simulink model "Example_2_Integral_Control_Mdl"  (Simulink 7.1)
settings: Solver=ode23s  StartTime=0.0  StopTime=5  RelTol=1e-3
values from neighbouring files (symbols this model uses):
  A = sys.a    [Example_2_Control.m]    (also in Example_2_Discretization.m; Example_2_Disturbance_Estimation.m; Example_2_Integral_Control.m; Example_2_Prediction_Observer.m)
  a_ramp = 0.05    [Example_2_Control.m]    (also in Example_2_Discretization.m; Example_2_Integral_Control.m; Example_2_Prediction_Observer.m; Example_2_Reduced_Order_Observer.m)
  a_sin = 0.1    [Example_2_Control.m]    (also in Example_2_Discretization.m; Example_2_Integral_Control.m; Example_2_Prediction_Observer.m; Example_2_Reduced_Order_Observer.m)
  B = sys.b    [Example_2_Control.m]    (also in Example_2_Discretization.m; Example_2_Disturbance_Estimation.m; Example_2_Integral_Control.m; Example_2_Prediction_Observer.m)
  B_w = sys_d.b    [Example_2_Control.m]    (also in Example_2_Discretization.m; Example_2_Disturbance_Estimation.m; Example_2_Integral_Control.m; Example_2_Prediction_Observer.m)
  C = sys.c    [Example_2_Control.m]    (also in Example_2_Discretization.m; Example_2_Disturbance_Estimation.m; Example_2_Integral_Control.m; Example_2_Prediction_Observer.m)
  h = T_r/N_r    [Example_2_Control.m]    (also in Example_2_Discretization.m; Example_2_Disturbance_Estimation.m; Example_2_Integral_Control.m; Example_2_Prediction_Observer.m)
  K = -K    [Example_2_Control.m]    (also in Example_2_Disturbance_Estimation.m; Example_2_Integral_Control.m = -K_aug(2:n_aug); Example_2_Reference_Tracking.m; Example_4_Active_Suspension_System.m)
  K_I = -K_aug(1)    [Example_2_Integral_Control.m]
  l_ramp = 0.05    [Example_2_Control.m]    (also in Example_2_Discretization.m; Example_2_Integral_Control.m; Example_2_Prediction_Observer.m; Example_2_Reduced_Order_Observer.m)
  l_sin = 5    [Example_2_Control.m]    (also in Example_2_Discretization.m; Example_2_Integral_Control.m; Example_2_Prediction_Observer.m; Example_2_Reduced_Order_Observer.m)
  N_x = N(1:n,:)    [Example_2_Integral_Control.m]    (also in Example_2_Reference_Tracking.m)
  v = 40/3.6    (= 11.1111111111)    [Example_2_Control.m]    (also in Example_2_Discretization.m; Example_2_Disturbance_Estimation.m; Example_2_Integral_Control.m; Example_2_Prediction_Observer.m)
  x_0 = [0; 0; 0; 0]    [Example_2_Analysis.m]    (also in Example_2_Control.m = [25*9.81/k_s; 0; 25*9.81/k_u; 0]; Example_2_Discretization.m = [25*9.81/k_s; 0; 25*9.81/k_u; 0]; Example_2_Disturbance_Estimation.m; Example_2_Integral_Control.m)
libraries: simulink x1
settings Model: Creator=d_goerges  LastModifiedBy=d_goerges
settings DataIOCC: Refine=10
settings OptimizationCC: InitFltsAndDblsToZero=off
settings DebuggingCC: FcnCallInpInsideContextMsg=Enable All  StrictBusMsg=ErrorLevel1
settings GRTTargetCC: CPPClassGenCompliant=off

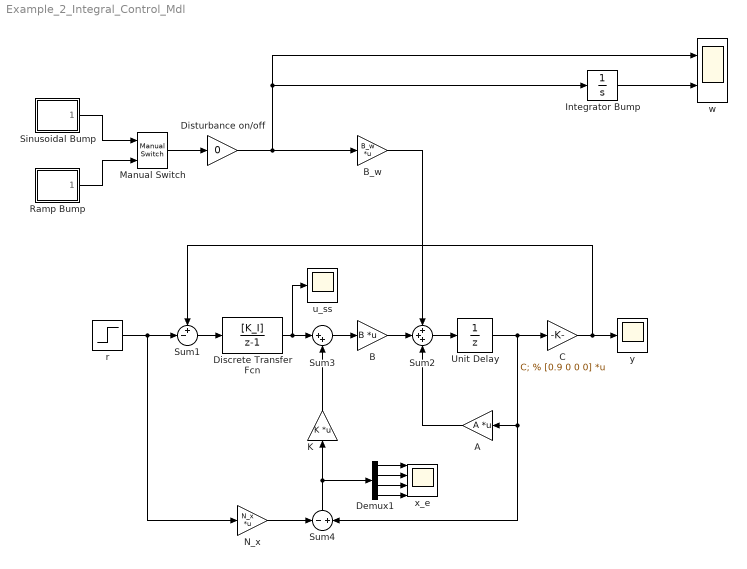
== system Example_2_Integral_Control_Mdl ==
  A : Gain  Orientation=left  Gain=A  Multiplication=Matrix(K*u)
  B : Gain  Gain=B  Multiplication=Matrix(K*u)
  B_w : Gain  Gain=B_w  Multiplication=Matrix(K*u)  SampleTime=h
  C : Gain  Gain=C; % [0.9 0 0 0]  Multiplication=Matrix(K*u)
  Demux1 : Demux
  Discrete Transfer Fcn : DiscreteTransferFcn  Numerator=[K_I]  Denominator=[1 -1]  SampleTime=h
  Disturbance on/off : Gain  Gain=0
  Integrator Bump : Integrator
  K : Gain  Orientation=up  Gain=K  Multiplication=Matrix(K*u)
  Manual Switch : simulink/Signal Routing/Manual Switch  sw=1  action=0  varsize=off
  N_x : Gain  Gain=N_x  Multiplication=Matrix(K*u)
  Ramp Bump : Subsystem
  Sinusoidal Bump : Subsystem
  Sum1 : Sum  Inputs=+-|
  Sum2 : Sum  Inputs=+++
  Sum3 : Sum  Inputs=|++
  Sum4 : Sum  Orientation=up  Inputs=-|+
  Unit Delay : UnitDelay  X0=x_0  SampleTime=h
  r : Step  After=0.02  SampleTime=0
  u_ss : Scope
  w : Scope  NumInputPorts=2
      settings: YMin=-5~-5  YMax=5~5  SaveName=ScopeData2
  x_e : Scope  NumInputPorts=4
      settings: YMin=-5~-5~-5~-5  YMax=5~5~5~5
  y : Scope
      settings: SaveName=ScopeData6
  wires:
  Sum2/1 -> Unit Delay/1
  C/1 -> y/1, Sum1/1
  Manual Switch/1 -> Disturbance on/off/1
  Unit Delay/1 -> C/1, A/1, Sum4/2
  Sinusoidal Bump/1(z_r_dot) -> Manual Switch/1
  Ramp Bump/1(z_r_dot) -> Manual Switch/2
  Integrator Bump/1 -> w/2
  Sum3/1 -> B/1
  r/1 -> N_x/1, Sum1/2
  B/1 -> Sum2/2
  A/1 -> Sum2/3
  Sum4/1 -> K/1, Demux1/1
  Sum1/1 -> Discrete Transfer Fcn/1
  Discrete Transfer Fcn/1 -> Sum3/1, u_ss/1
  K/1 -> Sum3/2
  B_w/1 -> Sum2/1
  N_x/1 -> Sum4/1
  Demux1/1 -> x_e/1
  Demux1/2 -> x_e/2
  Demux1/3 -> x_e/3
  Demux1/4 -> x_e/4
  Disturbance on/off/1 -> B_w/1, w/1, Integrator Bump/1

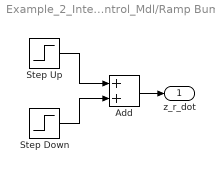
== system Example_2_Integral_Control_Mdl/Ramp Bump ==
  Add : Sum
  Step Down : Step  Time=l_ramp/v  After=-a_ramp/l_ramp*v  SampleTime=0
  Step Up : Step  Time=0  After=a_ramp/l_ramp*v  SampleTime=0
  z_r_dot : Outport
  wires:
  Step Up/1 -> Add/1
  Step Down/1 -> Add/2
  Add/1 -> z_r_dot/1

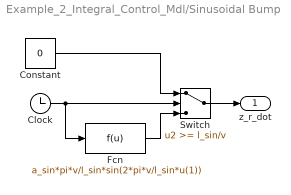
== system Example_2_Integral_Control_Mdl/Sinusoidal Bump ==
  Clock : Clock
  Constant : Constant  Value=0
  Fcn : Fcn  Expr=a_sin*pi*v/l_sin*sin(2*pi*v/l_sin*u(1))
  Switch : Switch  Threshold=l_sin/v
  z_r_dot : Outport
  wires:
  Switch/1 -> z_r_dot/1
  Fcn/1 -> Switch/3
  Constant/1 -> Switch/1
  Clock/1 -> Fcn/1, Switch/2
